simulink model "SF1"  (R2017b)
settings: Solver=VariableStepAuto  StartTime=0.0  StopTime=1  RelTol=1e-3
settings Model: Creator=Iman  LastModifiedBy=Iman

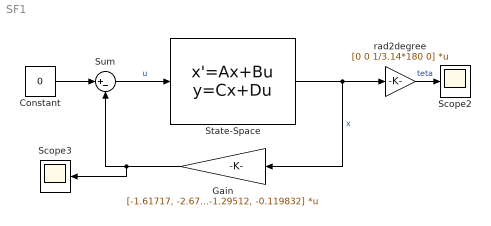
== system SF1 ==
  Constant : Constant  Value=0
  Gain : Gain  Gain=[-1.61717, -2.67843, -1.29512, -0.119832]  Multiplication=Matrix(K*u)
  Scope2 : Scope
  Scope3 : Scope
  State-Space : StateSpace  A="[0 1 0 0; 0,  -164.7, -1.5595,  4.52926;0 0 0 1;0, 3822.21, 112.493, -105.111]"  B=[0;102.59;0;-2417.31]  C=eye(4)  D=zeros(4,1)  InitialCondition=[0 0 0.01 0]
  Sum : Sum  Inputs=|+-
  rad2degree : Gain  Gain=[0 0 1/3.14*180 0]  Multiplication=Matrix(K*u)
  wires:
  Gain/1 -> Scope3/1, Sum/2
  Constant/1 -> Sum/1
  rad2degree/1 -> Scope2/1  "teta"
  State-Space/1 -> rad2degree/1, Gain/1  "x"
  Sum/1 -> State-Space/1  "u"
